simulink model "SOFC"  (R2021a)
settings: Solver=VariableStepAuto  StartTime=0.0  StopTime=10.0  RelTol=1e-3
settings Model: Creator=djoroya  LastModifiedBy=djoroya
settings OptimizationCC: BlockReduction=off  DefaultParameterBehavior=Inlined  BufferReuse=off

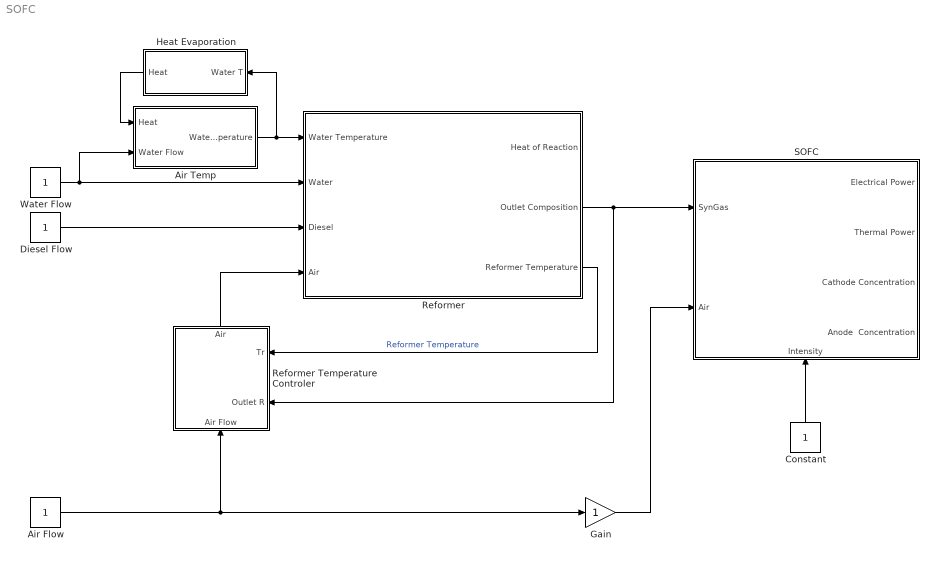
== system SOFC ==
  Air Flow : Constant
  Air Temp : Subsystem
  Constant : Constant
  Diesel Flow : Constant
  Gain : Gain
  Heat Evaporation : Subsystem
  Reformer : Subsystem
  Reformer Temperature Controler : Subsystem
      settings: PortSchema="{\"entries\":[{\"content\":{\"sides\":[{\"content\":{\"connectorIds\":[\"In1\",\"In2\"]},\"type\":\"ConnectorPlacement.EquallySpacedRectSide\",\"uuid\":\"f366bef7-1cbb-454c-ba22-5045f5dad993\"},{\"content\":{\"connectorIds\":[],\"side\":\"RIGHT\"},\"type\":\"ConnectorPlacement.EquallySpacedRectSide\",\"uuid\":\"c532895a-eea6-47ee-8799-b17744a19fa3\"},{\"content\":{\"connectorIds\":[\"Out1\"],\"side\":\"TOP\"},\"type\":\"ConnectorPlacement.EquallySpacedRectSide\",\"uuid\":\"b668778e-389b-4b28-b222-2d18ef70f538\"},{\"content\":{\"connectorIds\":[\"In3\"],\"side\":\"BOTTOM\"},\"type\":\"ConnectorPlacement.EquallySpacedRectSide\",\"uuid\":\"1611dce1-5d1a-4f48-9ab9-854e3377c643\"}]},\"type\":\"ConnectorPlacement.EquallySpacedConnector\",\"uuid\":\"ee861b9e-c999-44fa-90f8-d5c537479ed3\"}],\"packageUris\":[\"http://schema.mathworks.com/mf0/Connector/R2020b\"],\"version\":\"1.0\"}"
  SOFC : Subsystem
      settings: PortSchema="{\"entries\":[{\"content\":{\"sides\":[{\"content\":{\"connectorIds\":[\"In1\",\"In2\"]},\"type\":\"ConnectorPlacement.EquallySpacedRectSide\",\"uuid\":\"1940ef49-4b5a-4a2b-b4b2-e22fc2c3c082\"},{\"content\":{\"connectorIds\":[\"Out1\",\"Out2\",\"Out3\",\"Out4\"],\"side\":\"RIGHT\"},\"type\":\"ConnectorPlacement.EquallySpacedRectSide\",\"uuid\":\"6e4fcba8-b05e-4008-97af-823c00602f21\"},{\"content\":{\"connectorIds\":[],\"side\":\"TOP\"},\"type\":\"ConnectorPlacement.EquallySpacedRectSide\",\"uuid\":\"d1dbbd17-10ad-4348-9e67-987e9153d477\"},{\"content\":{\"connectorIds\":[\"In3\"],\"side\":\"BOTTOM\"},\"type\":\"ConnectorPlacement.EquallySpacedRectSide\",\"uuid\":\"c92de3b7-af8b-42ba-85d1-99583f405438\"}]},\"type\":\"ConnectorPlacement.EquallySpacedConnector\",\"uuid\":\"5036c0ee-5b5c-4b74-b95a-2adcd2a45d34\"}],\"packageUris\":[\"http://schema.mathworks.com/mf0/Connector/R2020b\"],\"version\":\"1.0\"}"
  Water Flow : Constant
  wires:
  Air Flow/1 -> Gain/1, Reformer Temperature Controler/3(Air Flow)
  Water Flow/1 -> Air Temp/2(Water Flow), Reformer/2(Water)
  Diesel Flow/1 -> Reformer/3(Diesel)
  Heat Evaporation/1("Heat ") -> Air Temp/1("Heat ")
  Air Temp/1(Water Temperature) -> Heat Evaporation/1(Water T), Reformer/1(Water Temperature)
  Constant/1 -> SOFC/3(Intensity)
  Gain/1 -> SOFC/2(Air)
  Reformer/2(Outlet Composition) -> SOFC/1(SynGas), Reformer Temperature Controler/2(Outlet R)
  Reformer/3(Reformer Temperature) -> Reformer Temperature Controler/1(Tr)  "Reformer Temperature"
  Reformer Temperature Controler/1(Air) -> Reformer/4(Air)

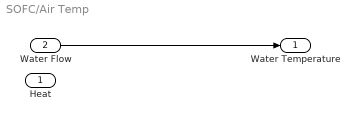
== system SOFC/Air Temp ==
  "Heat " : Inport
  Water Flow : Inport  Port=2
  Water Temperature : Outport
  wires:
  Water Flow/1 -> Water Temperature/1

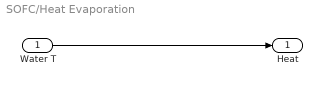
== system SOFC/Heat Evaporation ==
  Water T : Inport
  "Heat " : Outport
  wires:
  Water T/1 -> "Heat "/1

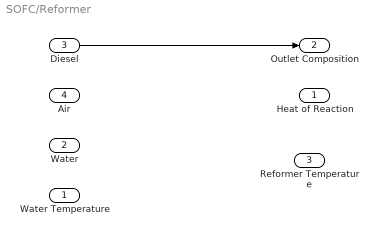
== system SOFC/Reformer ==
  Water Temperature : Inport
  Water : Inport  Port=2
  Diesel : Inport  Port=3
  Air : Inport  Port=4
  Heat of Reaction : Outport
  Outlet Composition : Outport  Port=2
  Reformer Temperature : Outport  Port=3
  wires:
  Diesel/1 -> Outlet Composition/1

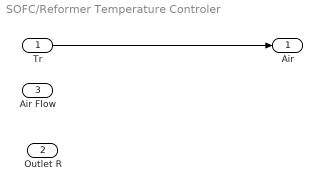
== system SOFC/Reformer Temperature Controler ==
  Tr : Inport
  Outlet R : Inport  Port=2
  Air Flow : Inport  Port=3
  Air : Outport
  wires:
  Tr/1 -> Air/1

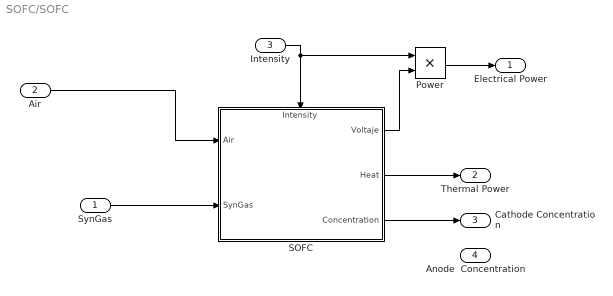
== system SOFC/SOFC ==
  SynGas : Inport
  Air : Inport  Port=2
  Intensity : Inport  Port=3
  Power : Product
  SOFC : Subsystem
      settings: PortSchema="{\"entries\":[{\"content\":{\"sides\":[{\"content\":{\"connectorIds\":[\"In1\",\"In2\"]},\"type\":\"ConnectorPlacement.EquallySpacedRectSide\",\"uuid\":\"f366bef7-1cbb-454c-ba22-5045f5dad993\"},{\"content\":{\"connectorIds\":[\"Out1\",\"Out2\",\"Out3\"],\"side\":\"RIGHT\"},\"type\":\"ConnectorPlacement.EquallySpacedRectSide\",\"uuid\":\"c532895a-eea6-47ee-8799-b17744a19fa3\"},{\"content\":{\"connectorIds\":[\"In3\"],\"side\":\"TOP\"},\"type\":\"ConnectorPlacement.EquallySpacedRectSide\",\"uuid\":\"b668778e-389b-4b28-b222-2d18ef70f538\"}]},\"type\":\"ConnectorPlacement.EquallySpacedConnector\",\"uuid\":\"ee861b9e-c999-44fa-90f8-d5c537479ed3\"}],\"packageUris\":[\"http://schema.mathworks.com/mf0/Connector/R2020b\"],\"version\":\"1.0\"}"
  Electrical Power : Outport
  Thermal Power : Outport  Port=2
  Cathode Concentration : Outport  Port=3
  Anode  Concentration : Outport  Port=4
  wires:
  SynGas/1 -> SOFC/2(SynGas)
  Air/1 -> SOFC/1(Air)
  Power/1 -> Electrical Power/1
  SOFC/1(Voltaje) -> Power/2
  SOFC/3(Concentration) -> Cathode Concentration/1
  SOFC/2(Heat) -> Thermal Power/1
  Intensity/1 -> SOFC/3(Intensity), Power/1

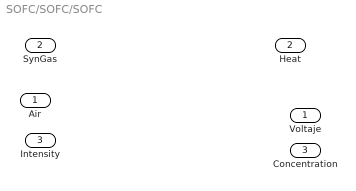
== system SOFC/SOFC/SOFC ==
  Air : Inport
  SynGas : Inport  Port=2
  Intensity : Inport  Port=3
  Voltaje : Outport
  Heat : Outport  Port=2
  Concentration : Outport  Port=3
